simulink model "AddTwoNumbers_Model"  (R2024b)
settings: Solver=VariableStepAuto  StartTime=0.0  StopTime=10.0  RelTol=1e-3
settings Model: Creator=Ahmad  LastModifiedBy=Ahmad

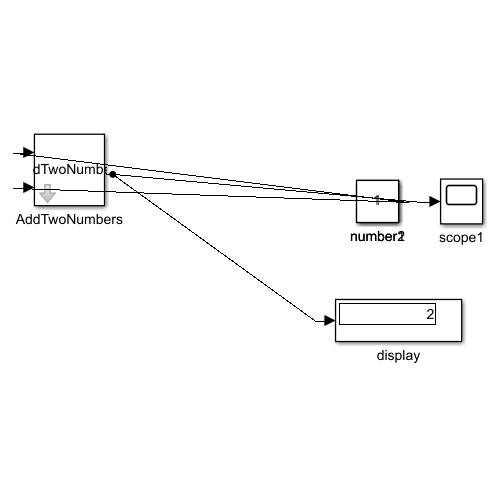
[thumbnail: Simulink's stored preview of the top-level diagram]
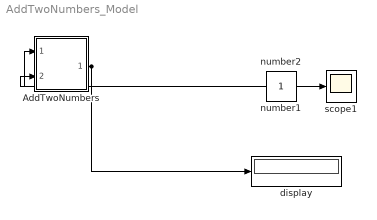
== system AddTwoNumbers_Model ==
  AddTwoNumbers : Subsystem  mask(AddTwoNumbersSubSystemBlock){}
      mask help: SubSystem Add two Numbers
      mask Display: disp("AddTwoNumbers")
  display : Display
  number1 : Constant
  number2 : Constant
  scope1 : Scope
  wires:
  number1/1 -> AddTwoNumbers/1(NumberOne)
  number2/1 -> AddTwoNumbers/2(NumberTwo)
  AddTwoNumbers/1(Summation) -> scope1/1, display/1

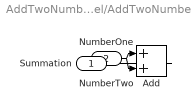
== system AddTwoNumbers_Model/AddTwoNumbers ==
  NumberOne : Inport
  NumberTwo : Inport  Port=2
  Add : Sum
  Summation : Outport
  wires:
  NumberOne/1 -> Add/1
  NumberTwo/1 -> Add/2
  Add/1 -> Summation/1
